simulink model "Xcvr_SSB_AM_2p5"  (Simulink 8.0)
settings: Solver=VariableStepDiscrete  SolverMode=SingleTasking  StartTime=0.0  StopTime=10  RelTol=1e-3
PreLoadFcn:
  | Fs=80e6;
  | 
  | phee=da_rom();
  | [phee_1,phee_2]=da_i2_rom();
  | 
  | Dcic=64;       % CIC decimation
  | Dfac=128;    % following DA filter decimation
  | N = 6;           %       (2^(N+1))=Dfac
  | Daudio=Dcic*Dfac;
  | Faudio=Fs/Daudio;
  | 
  | load info_filt_ssb_4
  | load Serial_Intfc_Stream_5
  | 
  | % AGC related
  | x=0.5:1/256:(1-1/256);
  | addr=(x-0.5)*256;
  | y=1./x;
values from neighbouring files (symbols this model uses):
  Serial_Interface = [0 0 0 0 0 0 0 0 0 0 0 0 ... (11390 elements, 2x5695)]    [Serial_Intfc_Stream_5.mat]
undefined symbols (not defined in the file or in its folder): get, sided, Two, xlipgetpartsetting
undefined symbols (not defined in the file): ssb_coef
libraries: xbsIndex_r4 x1307, dspsrcs4 x5, simulink x2, dspsigops x2, dspsnks4 x1
(part 10 of 11)

== system Xcvr_SSB_AM_2p5/RX Filters D=8192/Decimating Filter DC Optimized in Accumulator Plus Pipelined Stage Control. Improved dynamic  range. /D=2 Bit Serial Filter Core with Piplined RAM Based SR/ROM /Accumulator ==
  Xn + Xn-8 : Inport
  "Xn-1+ Xn-7 " : Inport  Port=2
  Xn-2 + Xn-6 : Inport  Port=3
  Xn-3 + Xn-5 : Inport  Port=4
  Xn-4 : Inport  Port=5
  Yn-2 : Inport  Port=6
  Yn-4 : Inport  Port=7
  Subtract : Inport  Port=8
  Clear : Inport  Port=9
  Round : Inport  Port=10
  AddSub : xbsIndex_r4/AddSub  mode=Addition  use_carryin=off  use_carryout=off  en=off  latency=0  precision=User Defined  arith_type="Signed  (2's comp)"  n_bits=24  bin_pt=0  quantization=Truncate  overflow=Wrap  dbl_ovrd=off  use_behavioral_HDL=off  hw_selection=Fabric  pipelined=off  use_rpm=on  block_type=addsub
      settings: block_version=9.2.00
  AddSub1 : xbsIndex_r4/AddSub  mode=Addition  use_carryin=off  use_carryout=off  en=off  latency=0  precision=User Defined  arith_type="Signed  (2's comp)"  n_bits=24  bin_pt=0  quantization=Truncate  overflow=Wrap  dbl_ovrd=off  use_behavioral_HDL=off  hw_selection=Fabric  pipelined=off  use_rpm=on  block_type=addsub
      settings: block_version=9.2.00
  Concat : xbsIndex_r4/Concat  num_inputs=8  dbl_ovrd=off  block_type=concat
      settings: block_version=9.2.00
  Convert : xbsIndex_r4/Convert  gui_display_data_type=Fixed-point  arith_type="Signed  (2's comp)"  n_bits=2  bin_pt=0  float_type=Single  exp_bits=8  fraction_bits=24  quantization=Truncate  overflow=Wrap  en=off  latency=0  dbl_ovrd=off  pipeline=off  block_type=convert
      settings: block_version=9.2.00
  ROM : xbsIndex_r4/ROM  depth=256  initVector=phee  distributed_mem=Block RAM  rst=off  init_reg=0  en=off  latency=1  gui_display_data_type=Fixed-point  arith_type="Signed  (2's comp)"  n_bits=13  bin_pt=0  preci_type=Single  exp_width=8  frac_width=24  dbl_ovrd=off  optimize=Area  use_rpm=on  block_type=sprom
      settings: block_version=9.2.00
  Register_M1 : xbsIndex_r4/Register  init=0  rst=on  en=off  dbl_ovrd=off  block_type=register
      settings: block_version=9.2.00
  Reinterpret1 : xbsIndex_r4/Reinterpret  force_arith_type=on  arith_type="Signed  (2's comp)"  force_bin_pt=on  bin_pt=0  block_type=reinterpret
      settings: infoedit="Changes signal type without altering the binary representation.   You can changed the signal between signed and unsigned, and relocate the binary point.<br><br>Hardware notes: In hardware this block costs nothing.<br><br>Example:  Suppose the input is 6 bits wide, signed, with 2 fractional bits, and the output is forced to unsigned with 0 fractional bits.  Then an input of -2.0 (1110.00 in binary 2's complement) becomes an output of 56 (111000 in binary)."  block_version=9.2.00
  Shift : xbsIndex_r4/Shift  shift_dir=Right  shift_bits=1  en=off  latency=0  precision=Full  arith_type="Signed  (2's comp)"  n_bits=18  bin_pt=0  quantization=Truncate  overflow=Wrap  dbl_ovrd=off  block_type=shift
      settings: block_version=9.2.00
  Shift1 : xbsIndex_r4/Shift  shift_dir=Left  shift_bits=10  en=off  latency=0  precision=User Defined  arith_type="Signed  (2's comp)"  n_bits=23  bin_pt=0  quantization=Truncate  overflow=Wrap  dbl_ovrd=off  block_type=shift
      settings: block_version=9.2.00
  Slice2 : xbsIndex_r4/Slice  nbits=21  boolean_output=off  mode=Lower Bit Location + Width  bit1=0  base1=MSB of Input  bit0=0  base0=LSB of Input  dbl_ovrd=off  block_type=slice
      settings: block_version=9.2.00
  Out1 : Outport
  wires:
  Subtract/1 -> Concat/1
  "Xn-1+ Xn-7 "/1 -> Concat/7
  Xn-2 + Xn-6/1 -> Concat/6
  Xn-3 + Xn-5/1 -> Concat/5
  Xn-4/1 -> Concat/4
  Yn-2/1 -> Concat/3
  Yn-4/1 -> Concat/2
  Xn + Xn-8/1 -> Concat/8
  Concat/1 -> ROM/1
  Clear/1 -> Register_M1/2
  Round/1 -> Convert/1
  ROM/1 -> Shift1/1
  Convert/1 -> AddSub1/2
  AddSub1/1 -> AddSub/2
  AddSub/1 -> Register_M1/1
  Reinterpret1/1 -> Out1/1
  Slice2/1 -> Reinterpret1/1
  Shift/1 -> AddSub/1
  Shift1/1 -> AddSub1/1
  Register_M1/1 -> Slice2/1, Shift/1

== system Xcvr_SSB_AM_2p5/RX Filters D=8192/Decimating Filter DC Optimized in Accumulator Plus Pipelined Stage Control. Improved dynamic  range. /D=2 Bit Serial Filter Core with Piplined RAM Based SR/SAD_1 ==
  A : Inport
  B : Inport  Port=2
  Clear : Inport  Port=3
  Full Adder : Subsystem
  Register : xbsIndex_r4/Register  init=0  rst=on  en=off  dbl_ovrd=off  block_type=register
      settings: block_version=9.2.00
  Sum : Outport
  wires:
  Full Adder/1(Sum) -> Sum/1
  Full Adder/2(Cout) -> Register/1
  Register/1 -> Full Adder/3(Cin)
  A/1 -> Full Adder/1(A)
  B/1 -> Full Adder/2(B)
  Clear/1 -> Register/2

== system Xcvr_SSB_AM_2p5/RX Filters D=8192/Decimating Filter DC Optimized in Accumulator Plus Pipelined Stage Control. Improved dynamic  range. /D=2 Bit Serial Filter Core with Piplined RAM Based SR/SAD_2 ==
  A : Inport
  B : Inport  Port=2
  Clear : Inport  Port=3
  Full Adder : Subsystem
  Register : xbsIndex_r4/Register  init=0  rst=on  en=off  dbl_ovrd=off  block_type=register
      settings: block_version=9.2.00
  Sum : Outport
  wires:
  Clear/1 -> Register/2
  B/1 -> Full Adder/2(B)
  A/1 -> Full Adder/1(A)
  Register/1 -> Full Adder/3(Cin)
  Full Adder/2(Cout) -> Register/1
  Full Adder/1(Sum) -> Sum/1

== system Xcvr_SSB_AM_2p5/RX Filters D=8192/Decimating Filter DC Optimized in Accumulator Plus Pipelined Stage Control. Improved dynamic  range. /D=2 Bit Serial Filter Core with Piplined RAM Based SR/SAD_3 ==
  A : Inport
  B : Inport  Port=2
  Clear : Inport  Port=3
  Full Adder : Subsystem
  Register : xbsIndex_r4/Register  init=0  rst=on  en=off  dbl_ovrd=off  block_type=register
      settings: block_version=9.2.00
  Sum : Outport
  wires:
  Full Adder/1(Sum) -> Sum/1
  Full Adder/2(Cout) -> Register/1
  Register/1 -> Full Adder/3(Cin)
  A/1 -> Full Adder/1(A)
  B/1 -> Full Adder/2(B)
  Clear/1 -> Register/2

== system Xcvr_SSB_AM_2p5/RX Filters D=8192/Decimating Filter DC Optimized in Accumulator Plus Pipelined Stage Control. Improved dynamic  range. /D=2 Bit Serial Filter Core with Piplined RAM Based SR/SAD_4 ==
  A : Inport
  B : Inport  Port=2
  Clear : Inport  Port=3
  Full Adder : Subsystem
  Register : xbsIndex_r4/Register  init=0  rst=on  en=off  dbl_ovrd=off  block_type=register
      settings: block_version=9.2.00
  Sum : Outport
  wires:
  Clear/1 -> Register/2
  B/1 -> Full Adder/2(B)
  A/1 -> Full Adder/1(A)
  Register/1 -> Full Adder/3(Cin)
  Full Adder/2(Cout) -> Register/1
  Full Adder/1(Sum) -> Sum/1

== system Xcvr_SSB_AM_2p5/RX Filters D=8192/Decimating Filter DC Optimized in Accumulator Plus Pipelined Stage Control. Improved dynamic  range. /D=2 Bit Serial Filter Core with Piplined RAM Based SR/SRA ==
  Par_In : Inport
  Shift : Inport  Port=2
  Delay : xbsIndex_r4/Delay  rst=off  infoeditControl=Selection of Reset will increase slice count due to use of real FFs and instead of SRLs  en=off  latency=1  dbl_ovrd=off  reg_retiming=off  block_type=delay
      settings: block_version=9.2.00
  Delay1 : xbsIndex_r4/Delay  rst=off  infoeditControl=Selection of Reset will increase slice count due to use of real FFs and instead of SRLs  en=off  latency=1  dbl_ovrd=off  reg_retiming=off  block_type=delay
      settings: block_version=9.2.00
  Mux : xbsIndex_r4/Mux  inputs=2  en=off  latency=0  precision=Full  arith_type=Unsigned  n_bits=16  bin_pt=14  quantization=Truncate  overflow=Wrap  dbl_ovrd=off  block_type=mux
      settings: block_version=9.2.00
  Shift1 : xbsIndex_r4/Shift  shift_dir=Right  shift_bits=1  en=off  latency=0  precision=Full  arith_type="Signed  (2's comp)"  n_bits=16  bin_pt=14  quantization=Truncate  overflow=Wrap  dbl_ovrd=off  block_type=shift
      settings: block_version=9.2.00
  Slice : xbsIndex_r4/Slice  nbits=1  boolean_output=on  mode=Lower Bit Location + Width  bit1=0  base1=MSB of Input  bit0=0  base0=LSB of Input  dbl_ovrd=off  block_type=slice
      settings: infoedit="Extracts a given range of bits from each input sample and presents it at the output.  The output type is ordinarily unsigned with binary point at zero, but can be Boolean when the slice is one bit wide.<P><P>Hardware notes: In hardware this block costs nothing."  block_version=9.2.00
  Ser_Out : Outport
  wires:
  Delay1/1 -> Ser_Out/1
  Slice/1 -> Delay1/1
  Shift/1 -> Mux/1
  Mux/1 -> Slice/1, Shift1/1
  Delay/1 -> Mux/3
  Shift1/1 -> Delay/1
  Par_In/1 -> Mux/2

== system Xcvr_SSB_AM_2p5/RX Filters D=8192/Decimating Filter DC Optimized in Accumulator Plus Pipelined Stage Control. Improved dynamic  range. /D=2 Bit Serial Filter Core with Piplined RAM Based SR/SRB ==
  Par_In : Inport
  Shift : Inport  Port=2
  Delay : xbsIndex_r4/Delay  rst=off  infoeditControl=Selection of Reset will increase slice count due to use of real FFs and instead of SRLs  en=off  latency=1  dbl_ovrd=off  reg_retiming=off  block_type=delay
      settings: block_version=9.2.00
  Delay1 : xbsIndex_r4/Delay  rst=off  infoeditControl=Selection of Reset will increase slice count due to use of real FFs and instead of SRLs  en=off  latency=1  dbl_ovrd=off  reg_retiming=off  block_type=delay
      settings: block_version=9.2.00
  Mux : xbsIndex_r4/Mux  inputs=2  en=off  latency=0  precision=Full  arith_type=Unsigned  n_bits=16  bin_pt=14  quantization=Truncate  overflow=Wrap  dbl_ovrd=off  block_type=mux
      settings: block_version=9.2.00
  Shift1 : xbsIndex_r4/Shift  shift_dir=Right  shift_bits=1  en=off  latency=0  precision=Full  arith_type="Signed  (2's comp)"  n_bits=16  bin_pt=14  quantization=Truncate  overflow=Wrap  dbl_ovrd=off  block_type=shift
      settings: block_version=9.2.00
  Slice : xbsIndex_r4/Slice  nbits=1  boolean_output=on  mode=Lower Bit Location + Width  bit1=0  base1=MSB of Input  bit0=0  base0=LSB of Input  dbl_ovrd=off  block_type=slice
      settings: infoedit="Extracts a given range of bits from each input sample and presents it at the output.  The output type is ordinarily unsigned with binary point at zero, but can be Boolean when the slice is one bit wide.<P><P>Hardware notes: In hardware this block costs nothing."  block_version=9.2.00
  Ser_Out : Outport
  wires:
  Delay1/1 -> Ser_Out/1
  Slice/1 -> Delay1/1
  Par_In/1 -> Mux/2
  Shift1/1 -> Delay/1
  Delay/1 -> Mux/3
  Mux/1 -> Shift1/1, Slice/1
  Shift/1 -> Mux/1

== system Xcvr_SSB_AM_2p5/RX Filters D=8192/Decimating Filter DC Optimized in Accumulator Plus Pipelined Stage Control. Improved dynamic  range. /D=2 Bit Serial Filter Core with Piplined RAM Based SR/SRC ==
  Par_In : Inport
  Shift : Inport  Port=2
  Delay : xbsIndex_r4/Delay  rst=off  infoeditControl=Selection of Reset will increase slice count due to use of real FFs and instead of SRLs  en=off  latency=1  dbl_ovrd=off  reg_retiming=off  block_type=delay
      settings: block_version=9.2.00
  Delay1 : xbsIndex_r4/Delay  rst=off  infoeditControl=Selection of Reset will increase slice count due to use of real FFs and instead of SRLs  en=off  latency=1  dbl_ovrd=off  reg_retiming=off  block_type=delay
      settings: block_version=9.2.00
  Mux : xbsIndex_r4/Mux  inputs=2  en=off  latency=0  precision=Full  arith_type=Unsigned  n_bits=16  bin_pt=14  quantization=Truncate  overflow=Wrap  dbl_ovrd=off  block_type=mux
      settings: block_version=9.2.00
  Shift1 : xbsIndex_r4/Shift  shift_dir=Right  shift_bits=1  en=off  latency=0  precision=Full  arith_type="Signed  (2's comp)"  n_bits=16  bin_pt=14  quantization=Truncate  overflow=Wrap  dbl_ovrd=off  block_type=shift
      settings: block_version=9.2.00
  Slice : xbsIndex_r4/Slice  nbits=1  boolean_output=on  mode=Lower Bit Location + Width  bit1=0  base1=MSB of Input  bit0=0  base0=LSB of Input  dbl_ovrd=off  block_type=slice
      settings: infoedit="Extracts a given range of bits from each input sample and presents it at the output.  The output type is ordinarily unsigned with binary point at zero, but can be Boolean when the slice is one bit wide.<P><P>Hardware notes: In hardware this block costs nothing."  block_version=9.2.00
  Ser_Out : Outport
  wires:
  Delay1/1 -> Ser_Out/1
  Slice/1 -> Delay1/1
  Shift/1 -> Mux/1
  Mux/1 -> Slice/1, Shift1/1
  Delay/1 -> Mux/3
  Shift1/1 -> Delay/1
  Par_In/1 -> Mux/2

== system Xcvr_SSB_AM_2p5/RX Filters D=8192/Decimating Filter DC Optimized in Accumulator Plus Pipelined Stage Control. Improved dynamic  range. /D=2 Bit Serial Filter Core with Piplined RAM Based SR/Timing/Control1 ==
  Start : Inport
  AddSub : xbsIndex_r4/AddSub  mode=Addition  use_carryin=off  use_carryout=off  en=off  latency=0  precision=User Defined  arith_type=Unsigned  n_bits=5  bin_pt=0  quantization=Truncate  overflow=Wrap  dbl_ovrd=off  use_behavioral_HDL=off  hw_selection=Fabric  pipelined=off  use_rpm=on  block_type=addsub
      settings: block_version=9.2.00
  Constant : xbsIndex_r4/Constant  const=26  gui_display_data_type=Fixed-point  arith_type=Unsigned  n_bits=5  bin_pt=0  preci_type=Single  exp_width=8  frac_width=24  explicit_period=off  period=1  equ=P=C  opselect=C  inp2=PCIN>>17  opr=+  inp1=P  carry=CIN  dbl_ovrd=off  block_type=constant
      settings: block_version=9.2.00
  Constant1 : xbsIndex_r4/Constant  const=1  gui_display_data_type=Fixed-point  arith_type=Unsigned  n_bits=5  bin_pt=0  preci_type=Single  exp_width=8  frac_width=24  explicit_period=off  period=1  equ=P=C  opselect=C  inp2=PCIN>>17  opr=+  inp1=P  carry=CIN  dbl_ovrd=off  block_type=constant
      settings: block_version=9.2.00
  Constant12 : xbsIndex_r4/Constant  const=2  gui_display_data_type=Fixed-point  arith_type=Unsigned  n_bits=5  bin_pt=0  preci_type=Single  exp_width=8  frac_width=24  explicit_period=off  period=1  equ=P=C  opselect=C  inp2=PCIN>>17  opr=+  inp1=P  carry=CIN  dbl_ovrd=off  block_type=constant
      settings: block_version=9.2.00
  Constant2 : xbsIndex_r4/Constant  const=0  gui_display_data_type=Fixed-point  arith_type=Unsigned  n_bits=5  bin_pt=0  preci_type=Single  exp_width=8  frac_width=24  explicit_period=off  period=1  equ=P=C  opselect=C  inp2=PCIN>>17  opr=+  inp1=P  carry=CIN  dbl_ovrd=off  block_type=constant
      settings: block_version=9.2.00
  Constant3 : xbsIndex_r4/Constant  const=0  gui_display_data_type=Fixed-point  arith_type=Unsigned  n_bits=5  bin_pt=0  preci_type=Single  exp_width=8  frac_width=24  explicit_period=off  period=1  equ=P=C  opselect=C  inp2=PCIN>>17  opr=+  inp1=P  carry=CIN  dbl_ovrd=off  block_type=constant
      settings: block_version=9.2.00
  Constant4 : xbsIndex_r4/Constant  const=1  gui_display_data_type=Fixed-point  arith_type=Unsigned  n_bits=5  bin_pt=0  preci_type=Single  exp_width=8  frac_width=24  explicit_period=off  period=1  equ=P=C  opselect=C  inp2=PCIN>>17  opr=+  inp1=P  carry=CIN  dbl_ovrd=off  block_type=constant
      settings: block_version=9.2.00
  Constant5 : xbsIndex_r4/Constant  const=25  gui_display_data_type=Fixed-point  arith_type=Unsigned  n_bits=5  bin_pt=0  preci_type=Single  exp_width=8  frac_width=24  explicit_period=off  period=1  equ=P=C  opselect=C  inp2=PCIN>>17  opr=+  inp1=P  carry=CIN  dbl_ovrd=off  block_type=constant
      settings: block_version=9.2.00
  Constant6 : xbsIndex_r4/Constant  const=23  gui_display_data_type=Fixed-point  arith_type=Unsigned  n_bits=5  bin_pt=0  preci_type=Single  exp_width=8  frac_width=24  explicit_period=off  period=1  equ=P=C  opselect=C  inp2=PCIN>>17  opr=+  inp1=P  carry=CIN  dbl_ovrd=off  block_type=constant
      settings: block_version=9.2.00
  Constant7 : xbsIndex_r4/Constant  const=2-1  gui_display_data_type=Fixed-point  arith_type=Unsigned  n_bits=5  bin_pt=0  preci_type=Single  exp_width=8  frac_width=24  explicit_period=off  period=1  equ=P=C  opselect=C  inp2=PCIN>>17  opr=+  inp1=P  carry=CIN  dbl_ovrd=off  block_type=constant
      settings: block_version=9.2.00
  Constant8 : xbsIndex_r4/Constant  const=21  gui_display_data_type=Fixed-point  arith_type=Unsigned  n_bits=5  bin_pt=0  preci_type=Single  exp_width=8  frac_width=24  explicit_period=off  period=1  equ=P=C  opselect=C  inp2=PCIN>>17  opr=+  inp1=P  carry=CIN  dbl_ovrd=off  block_type=constant
      settings: block_version=9.2.00
  Constant9 : xbsIndex_r4/Constant  const=23  gui_display_data_type=Fixed-point  arith_type=Unsigned  n_bits=5  bin_pt=0  preci_type=Single  exp_width=8  frac_width=24  explicit_period=off  period=1  equ=P=C  opselect=C  inp2=PCIN>>17  opr=+  inp1=P  carry=CIN  dbl_ovrd=off  block_type=constant
      settings: block_version=9.2.00
  Delay : xbsIndex_r4/Delay  rst=off  infoeditControl=Selection of Reset will increase slice count due to use of real FFs and instead of SRLs  en=off  latency=1  dbl_ovrd=off  reg_retiming=off  block_type=delay
      settings: block_version=9.2.00
  Logical : xbsIndex_r4/Logical  logical_function=AND  inputs=2  en=off  latency=0  precision=Full  arith_type=Unsigned  n_bits=16  bin_pt=0  align_bp=on  dbl_ovrd=off  block_type=logical
      settings: block_version=9.2.00
  Mux : xbsIndex_r4/Mux  inputs=2  en=off  latency=0  precision=Full  arith_type=Unsigned  n_bits=16  bin_pt=14  quantization=Truncate  overflow=Wrap  dbl_ovrd=off  block_type=mux
      settings: block_version=9.2.00
  Relational{,2..4,7,10} (6 alike) : xbsIndex_r4/Relational  mode=a=b  en=off  latency=0  dbl_ovrd=off  block_type=relational
      settings: block_version=9.2.00
  Relational1 : xbsIndex_r4/Relational  mode=a>b  en=off  latency=0  dbl_ovrd=off  block_type=relational
      settings: block_version=9.2.00
  Relational5 : xbsIndex_r4/Relational  mode=a>=b  en=off  latency=0  dbl_ovrd=off  block_type=relational
      settings: block_version=9.2.00
  Relational6 : xbsIndex_r4/Relational  mode=a<=b  en=off  latency=0  dbl_ovrd=off  block_type=relational
      settings: block_version=9.2.00
  S-R FF1 : Subsystem
  Run : Outport
  Clear_Adder : Outport  Port=2
  Strobe : Outport  Port=3
  Subtract : Outport  Port=4
  SR Enable : Outport  Port=5
  Round : Outport  Port=6
  Clear_Acc : Outport  Port=7
  Valid : Outport  Port=8
  wires:
  Relational4/1 -> Subtract/1
  Relational1/1 -> Run/1
  Delay/1 -> Relational5/1, Relational6/1, Relational7/1, Relational3/1, Relational2/1, AddSub/1, Relational/1, Relational1/1, Relational10/1, Relational4/1
  Relational/1 -> S-R FF1/2(Reset), Valid/1
  Constant/1 -> Relational/2
  S-R FF1/1(Q) -> Mux/1
  Start/1 -> S-R FF1/1(Set)
  Mux/1 -> Delay/1
  AddSub/1 -> Mux/3
  Constant1/1 -> AddSub/2
  Constant2/1 -> Mux/2
  Constant3/1 -> Relational1/2
  Constant4/1 -> Relational2/2
  Relational2/1 -> Clear_Adder/1
  Constant5/1 -> Relational3/2
  Relational3/1 -> Strobe/1
  Constant6/1 -> Relational4/2
  Constant7/1 -> Relational5/2
  Constant8/1 -> Relational6/2
  Relational5/1 -> Logical/1
  Relational6/1 -> Logical/2
  Logical/1 -> SR Enable/1
  Constant9/1 -> Relational7/2
  Relational7/1 -> Round/1
  Constant12/1 -> Relational10/2
  Relational10/1 -> Clear_Acc/1

== system Xcvr_SSB_AM_2p5/RX Filters D=8192/Decimating Filter DC Optimized in Accumulator Plus Pipelined Stage Control. Improved dynamic  range. /Stage Control with Pipe/Stage_Control ==
  Concat : xbsIndex_r4/Concat  num_inputs=3  dbl_ovrd=off  block_type=concat
      settings: block_version=9.2.00
  Counter : xbsIndex_r4/Counter  cnt_type=Free Running  cnt_to=Inf  operation=Up  start_count=0  cnt_by_val=1  arith_type=Unsigned  n_bits=7  bin_pt=0  load_pin=off  rst=off  en=off  explicit_period=on  period=64/Fs  dbl_ovrd=off  use_behavioral_HDL=off  implementation=Fabric  use_rpm=off  block_type=counter
      settings: block_version=9.2.00
  Logical : xbsIndex_r4/Logical  logical_function=NAND  inputs=7  en=off  latency=0  precision=Full  arith_type=Unsigned  n_bits=16  bin_pt=0  align_bp=on  dbl_ovrd=off  block_type=logical
      settings: block_version=9.2.00
  Priority_Encoder : Subsystem
  bit_0 : xbsIndex_r4/Slice  nbits=1  boolean_output=on  mode=Lower Bit Location + Width  bit1=0  base1=MSB of Input  bit0=0  base0=LSB of Input  dbl_ovrd=off  block_type=slice
      settings: infoedit="Extracts a given range of bits from each input sample and presents it at the output.  The output type is ordinarily unsigned with binary point at zero, but can be Boolean when the slice is one bit wide.<P><P>Hardware notes: In hardware this block costs nothing."  block_version=9.2.00
  bit_1 : xbsIndex_r4/Slice  nbits=1  boolean_output=on  mode=Lower Bit Location + Width  bit1=0  base1=MSB of Input  bit0=1  base0=LSB of Input  dbl_ovrd=off  block_type=slice
      settings: infoedit="Extracts a given range of bits from each input sample and presents it at the output.  The output type is ordinarily unsigned with binary point at zero, but can be Boolean when the slice is one bit wide.<P><P>Hardware notes: In hardware this block costs nothing."  block_version=9.2.00
  bit_2 : xbsIndex_r4/Slice  nbits=1  boolean_output=on  mode=Lower Bit Location + Width  bit1=0  base1=MSB of Input  bit0=2  base0=LSB of Input  dbl_ovrd=off  block_type=slice
      settings: infoedit="Extracts a given range of bits from each input sample and presents it at the output.  The output type is ordinarily unsigned with binary point at zero, but can be Boolean when the slice is one bit wide.<P><P>Hardware notes: In hardware this block costs nothing."  block_version=9.2.00
  bit_3 : xbsIndex_r4/Slice  nbits=1  boolean_output=on  mode=Lower Bit Location + Width  bit1=0  base1=MSB of Input  bit0=3  base0=LSB of Input  dbl_ovrd=off  block_type=slice
      settings: infoedit="Extracts a given range of bits from each input sample and presents it at the output.  The output type is ordinarily unsigned with binary point at zero, but can be Boolean when the slice is one bit wide.<P><P>Hardware notes: In hardware this block costs nothing."  block_version=9.2.00
  bit_4 : xbsIndex_r4/Slice  nbits=1  boolean_output=on  mode=Lower Bit Location + Width  bit1=0  base1=MSB of Input  bit0=4  base0=LSB of Input  dbl_ovrd=off  block_type=slice
      settings: infoedit="Extracts a given range of bits from each input sample and presents it at the output.  The output type is ordinarily unsigned with binary point at zero, but can be Boolean when the slice is one bit wide.<P><P>Hardware notes: In hardware this block costs nothing."  block_version=9.2.00
  bit_5 : xbsIndex_r4/Slice  nbits=1  boolean_output=on  mode=Lower Bit Location + Width  bit1=0  base1=MSB of Input  bit0=5  base0=LSB of Input  dbl_ovrd=off  block_type=slice
      settings: infoedit="Extracts a given range of bits from each input sample and presents it at the output.  The output type is ordinarily unsigned with binary point at zero, but can be Boolean when the slice is one bit wide.<P><P>Hardware notes: In hardware this block costs nothing."  block_version=9.2.00
  bit_6 : xbsIndex_r4/Slice  nbits=1  boolean_output=on  mode=Lower Bit Location + Width  bit1=0  base1=MSB of Input  bit0=6  base0=LSB of Input  dbl_ovrd=off  block_type=slice
      settings: infoedit="Extracts a given range of bits from each input sample and presents it at the output.  The output type is ordinarily unsigned with binary point at zero, but can be Boolean when the slice is one bit wide.<P><P>Hardware notes: In hardware this block costs nothing."  block_version=9.2.00
  Write_OK : Outport
  Filt_Stage : Outport  Port=2
  wires:
  bit_0/1 -> Priority_Encoder/7(In7), Logical/7
  bit_1/1 -> Priority_Encoder/6(In6), Logical/6
  bit_2/1 -> Priority_Encoder/5(In5), Logical/5
  bit_3/1 -> Priority_Encoder/4(In4), Logical/4
  bit_4/1 -> Priority_Encoder/3(In3), Logical/3
  bit_5/1 -> Priority_Encoder/2(In2), Logical/2
  bit_6/1 -> Priority_Encoder/1(In1), Logical/1
  Counter/1 -> bit_6/1, bit_0/1, bit_1/1, bit_2/1, bit_3/1, bit_4/1, bit_5/1
  Priority_Encoder/2(Out2) -> Concat/2
  Priority_Encoder/1(Out1) -> Concat/3
  Priority_Encoder/3(Out3) -> Concat/1
  Logical/1 -> Write_OK/1  "Write_OK"
  Concat/1 -> Filt_Stage/1  "Filt_Stage"

== system Xcvr_SSB_AM_2p5/SSB / AM Mod_Demod WCS/128 Tap FIR with  Writable Coefficient Store/Information_Filter_Transient_Suppressor/N_Sample_One_Shot ==
  In : Inport
  Counter : xbsIndex_r4/Counter  cnt_type=Free Running  cnt_to=Inf  operation=Up  start_count=0  cnt_by_val=1  arith_type=Unsigned  n_bits=8  bin_pt=0  load_pin=off  rst=on  en=off  explicit_period=off  period=1  dbl_ovrd=off  use_behavioral_HDL=off  implementation=Fabric  block_type=counter
      settings: block_version=12.1
  Inverter : xbsIndex_r4/Inverter  en=off  latency=0  dbl_ovrd=off  block_type=inv
      settings: block_version=12.1
  Logical : xbsIndex_r4/Logical  logical_function=OR  inputs=2  en=off  latency=0  precision=Full  arith_type=Unsigned  n_bits=16  bin_pt=0  align_bp=on  dbl_ovrd=off  block_type=logical
      settings: block_version=12.1
  N : xbsIndex_r4/Constant  const=N  gui_display_data_type=Fixed-point  arith_type=Unsigned  n_bits=8  bin_pt=0  preci_type=Single  exp_width=8  frac_width=24  explicit_period=off  period=1  equ=P=C  opselect=C  inp2=PCIN>>17  opr=+  inp1=P  carry=CIN  dbl_ovrd=off  block_type=constant
      settings: block_version=12.1
  Register : xbsIndex_r4/Register  init=0  rst=on  en=off  dbl_ovrd=off  block_type=register
      settings: block_version=12.1
  Relational : xbsIndex_r4/Relational  mode=a=b  en=off  latency=0  dbl_ovrd=off  block_type=relational
      settings: block_version=12.1
  Out : Outport
  wires:
  Logical/1 -> Register/1, Out/1
  Register/1 -> Logical/2, Inverter/1
  In/1 -> Logical/1
  Counter/1 -> Relational/1
  N/1 -> Relational/2
  Relational/1 -> Register/2
  Inverter/1 -> Counter/1

== system Xcvr_SSB_AM_2p5/Serial Interface1/Serial_in_Parallel_out/Serial2Par/Subsystem ==
  Sin : Inport
  Ena : Inport  Port=2
  Concat : xbsIndex_r4/Concat  num_inputs=8  dbl_ovrd=off  block_type=concat
      settings: block_version=9.2.00
  Register{1..8} (8 alike) : xbsIndex_r4/Register  init=0  rst=off  en=on  dbl_ovrd=off  block_type=register
      settings: block_version=9.2.00
  Out_8b : Outport
  Sout : Outport  Port=2
  wires:
  Ena/1 -> Register8/2, Register7/2, Register6/2, Register5/2, Register4/2, Register3/2, Register2/2, Register1/2
  Register2/1 -> Register3/1, Concat/7
  Register3/1 -> Register4/1, Concat/6
  Register4/1 -> Register5/1, Concat/5
  Register5/1 -> Register6/1, Concat/4
  Register6/1 -> Register7/1, Concat/3
  Register7/1 -> Register8/1, Concat/2
  Register8/1 -> Concat/1, Sout/1
  Concat/1 -> Out_8b/1
  Register1/1 -> Concat/8, Register2/1
  Sin/1 -> Register1/1

== system Xcvr_SSB_AM_2p5/Serial Interface1/Serial_in_Parallel_out/Serial2Par/Subsystem1 ==
  Sin : Inport
  Ena : Inport  Port=2
  Concat : xbsIndex_r4/Concat  num_inputs=8  dbl_ovrd=off  block_type=concat
      settings: block_version=9.2.00
  Register{1..8} (8 alike) : xbsIndex_r4/Register  init=0  rst=off  en=on  dbl_ovrd=off  block_type=register
      settings: block_version=9.2.00
  Out_8b : Outport
  Sout : Outport  Port=2
  wires:
  Sin/1 -> Register1/1
  Concat/1 -> Out_8b/1
  Register8/1 -> Sout/1, Concat/1
  Register7/1 -> Concat/2, Register8/1
  Register6/1 -> Concat/3, Register7/1
  Register5/1 -> Concat/4, Register6/1
  Register4/1 -> Concat/5, Register5/1
  Register3/1 -> Concat/6, Register4/1
  Register2/1 -> Concat/7, Register3/1
  Register1/1 -> Concat/8, Register2/1
  Ena/1 -> Register2/2, Register3/2, Register4/2, Register5/2, Register6/2, Register7/2, Register8/2, Register1/2

== system Xcvr_SSB_AM_2p5/Serial Interface1/Serial_in_Parallel_out/Serial2Par/Subsystem2 ==
  Sin : Inport
  Ena : Inport  Port=2
  Concat : xbsIndex_r4/Concat  num_inputs=8  dbl_ovrd=off  block_type=concat
      settings: block_version=9.2.00
  Register{1..8} (8 alike) : xbsIndex_r4/Register  init=0  rst=off  en=on  dbl_ovrd=off  block_type=register
      settings: block_version=9.2.00
  Out_8b : Outport
  Sout : Outport  Port=2
  wires:
  Ena/1 -> Register1/2, Register8/2, Register7/2, Register6/2, Register5/2, Register4/2, Register3/2, Register2/2
  Register1/1 -> Register2/1, Concat/8
  Register2/1 -> Register3/1, Concat/7
  Register3/1 -> Register4/1, Concat/6
  Register4/1 -> Register5/1, Concat/5
  Register5/1 -> Register6/1, Concat/4
  Register6/1 -> Register7/1, Concat/3
  Register7/1 -> Register8/1, Concat/2
  Register8/1 -> Concat/1, Sout/1
  Concat/1 -> Out_8b/1
  Sin/1 -> Register1/1

== system Xcvr_SSB_AM_2p5/Serial Interface1/Serial_in_Parallel_out/Serial2Par/Subsystem3 ==
  Sin : Inport
  Ena : Inport  Port=2
  Concat : xbsIndex_r4/Concat  num_inputs=8  dbl_ovrd=off  block_type=concat
      settings: block_version=9.2.00
  Register{1..8} (8 alike) : xbsIndex_r4/Register  init=0  rst=off  en=on  dbl_ovrd=off  block_type=register
      settings: block_version=9.2.00
  Out_8b : Outport
  Sout : Outport  Port=2
  wires:
  Sin/1 -> Register1/1
  Concat/1 -> Out_8b/1
  Register8/1 -> Sout/1, Concat/1
  Register7/1 -> Concat/2, Register8/1
  Register6/1 -> Concat/3, Register7/1
  Register5/1 -> Concat/4, Register6/1
  Register4/1 -> Concat/5, Register5/1
  Register3/1 -> Concat/6, Register4/1
  Register2/1 -> Concat/7, Register3/1
  Register1/1 -> Concat/8, Register2/1
  Ena/1 -> Register2/2, Register3/2, Register4/2, Register5/2, Register6/2, Register7/2, Register8/2, Register1/2

== system Xcvr_SSB_AM_2p5/TX Filters I=8192/Control/Stage_Control/Priority_Encoder ==
  In1 : Inport
  In2 : Inport  Port=2
  In3 : Inport  Port=3
  In4 : Inport  Port=4
  In5 : Inport  Port=5
  In6 : Inport  Port=6
  In7 : Inport  Port=7
  Inverter{,1..6} (7 alike) : xbsIndex_r4/Inverter  en=off  latency=0  dbl_ovrd=off  block_type=inv
      settings: block_version=9.2.00
  Logical : xbsIndex_r4/Logical  logical_function=AND  inputs=4  en=off  latency=0  precision=Full  arith_type=Unsigned  n_bits=16  bin_pt=0  align_bp=on  dbl_ovrd=off  block_type=logical
      settings: block_version=9.2.00
  Logical1 : xbsIndex_r4/Logical  logical_function=NOR  inputs=4  en=off  latency=0  precision=Full  arith_type=Unsigned  n_bits=16  bin_pt=0  align_bp=on  dbl_ovrd=off  block_type=logical
      settings: block_version=9.2.00
  Logical2 : xbsIndex_r4/Logical  logical_function=AND  inputs=3  en=off  latency=0  precision=Full  arith_type=Unsigned  n_bits=16  bin_pt=0  align_bp=on  dbl_ovrd=off  block_type=logical
      settings: block_version=9.2.00
  Logical3 : xbsIndex_r4/Logical  logical_function=AND  inputs=2  en=off  latency=0  precision=Full  arith_type=Unsigned  n_bits=16  bin_pt=0  align_bp=on  dbl_ovrd=off  block_type=logical
      settings: block_version=9.2.00
  Logical4 : xbsIndex_r4/Logical  logical_function=AND  inputs=3  en=off  latency=0  precision=Full  arith_type=Unsigned  n_bits=16  bin_pt=0  align_bp=on  dbl_ovrd=off  block_type=logical
      settings: block_version=9.2.00
  Logical5 : xbsIndex_r4/Logical  logical_function=AND  inputs=3  en=off  latency=0  precision=Full  arith_type=Unsigned  n_bits=16  bin_pt=0  align_bp=on  dbl_ovrd=off  block_type=logical
      settings: block_version=9.2.00
  Logical6 : xbsIndex_r4/Logical  logical_function=NOR  inputs=4  en=off  latency=0  precision=Full  arith_type=Unsigned  n_bits=16  bin_pt=0  align_bp=on  dbl_ovrd=off  block_type=logical
      settings: block_version=9.2.00
  Logical7 : xbsIndex_r4/Logical  logical_function=NOR  inputs=4  en=off  latency=0  precision=Full  arith_type=Unsigned  n_bits=16  bin_pt=0  align_bp=on  dbl_ovrd=off  block_type=logical
      settings: block_version=9.2.00
  Out1 : Outport
  Out2 : Outport  Port=2
  Out3 : Outport  Port=3
  wires:
  Logical7/1 -> Out3/1
  Logical6/1 -> Out2/1
  In7/1 -> Inverter6/1
  Logical1/1 -> Out1/1
  In3/1 -> Inverter2/1
  In1/1 -> Inverter/1
  Inverter3/1 -> Logical7/1
  Inverter4/1 -> Logical3/1, Logical7/2
  Inverter6/1 -> Logical1/4, Logical6/4, Logical7/4
  Inverter5/1 -> Logical7/3, Logical6/3
  Inverter1/1 -> Logical4/1
  Inverter2/1 -> Logical5/1, Logical2/1
  In6/1 -> Logical3/2, Logical2/3, Logical/4, Inverter5/1
  In5/1 -> Logical5/3, Logical4/3, Inverter4/1
  In4/1 -> Logical5/2, Logical4/2, Logical2/2, Logical/3, Inverter3/1
  In2/1 -> Logical/2, Inverter1/1
  Logical5/1 -> Logical6/2
  Logical4/1 -> Logical6/1
  Logical3/1 -> Logical1/3
  Logical2/1 -> Logical1/2
  Logical/1 -> Logical1/1
  Inverter/1 -> Logical/1

== system Xcvr_SSB_AM_2p5/TX Filters I=8192/Interp_Core/RAM Based SR/Bit-Extraction ==
  In1 : Inport
  B0 : xbsIndex_r4/Slice  nbits=1  boolean_output=on  mode=Lower Bit Location + Width  bit1=0  base1=MSB of Input  bit0=0  base0=LSB of Input  dbl_ovrd=off  block_type=slice
      settings: infoedit="Extracts a given range of bits from each input sample and presents it at the output.  The output type is ordinarily unsigned with binary point at zero, but can be Boolean when the slice is one bit wide.<P><P>Hardware notes: In hardware this block costs nothing."  block_version=9.2.00
  B1 : xbsIndex_r4/Slice  nbits=1  boolean_output=on  mode=Lower Bit Location + Width  bit1=0  base1=MSB of Input  bit0=1  base0=LSB of Input  dbl_ovrd=off  block_type=slice
      settings: infoedit="Extracts a given range of bits from each input sample and presents it at the output.  The output type is ordinarily unsigned with binary point at zero, but can be Boolean when the slice is one bit wide.<P><P>Hardware notes: In hardware this block costs nothing."  block_version=9.2.00
  B2 : xbsIndex_r4/Slice  nbits=1  boolean_output=on  mode=Lower Bit Location + Width  bit1=0  base1=MSB of Input  bit0=2  base0=LSB of Input  dbl_ovrd=off  block_type=slice
      settings: infoedit="Extracts a given range of bits from each input sample and presents it at the output.  The output type is ordinarily unsigned with binary point at zero, but can be Boolean when the slice is one bit wide.<P><P>Hardware notes: In hardware this block costs nothing."  block_version=9.2.00
  B3 : xbsIndex_r4/Slice  nbits=1  boolean_output=on  mode=Lower Bit Location + Width  bit1=0  base1=MSB of Input  bit0=3  base0=LSB of Input  dbl_ovrd=off  block_type=slice
      settings: infoedit="Extracts a given range of bits from each input sample and presents it at the output.  The output type is ordinarily unsigned with binary point at zero, but can be Boolean when the slice is one bit wide.<P><P>Hardware notes: In hardware this block costs nothing."  block_version=9.2.00
  B4 : xbsIndex_r4/Slice  nbits=1  boolean_output=on  mode=Lower Bit Location + Width  bit1=0  base1=MSB of Input  bit0=4  base0=LSB of Input  dbl_ovrd=off  block_type=slice
      settings: infoedit="Extracts a given range of bits from each input sample and presents it at the output.  The output type is ordinarily unsigned with binary point at zero, but can be Boolean when the slice is one bit wide.<P><P>Hardware notes: In hardware this block costs nothing."  block_version=9.2.00
  B5 : xbsIndex_r4/Slice  nbits=1  boolean_output=on  mode=Lower Bit Location + Width  bit1=0  base1=MSB of Input  bit0=5  base0=LSB of Input  dbl_ovrd=off  block_type=slice
      settings: infoedit="Extracts a given range of bits from each input sample and presents it at the output.  The output type is ordinarily unsigned with binary point at zero, but can be Boolean when the slice is one bit wide.<P><P>Hardware notes: In hardware this block costs nothing."  block_version=9.2.00
  b0 : Outport
  b1 : Outport  Port=2
  b2 : Outport  Port=3
  b3 : Outport  Port=4
  b4 : Outport  Port=5
  b5 : Outport  Port=6
  wires:
  B5/1 -> b5/1
  B4/1 -> b4/1
  B3/1 -> b3/1
  B2/1 -> b2/1
  B1/1 -> b1/1
  B0/1 -> b0/1
  In1/1 -> B3/1, B0/1, B1/1, B2/1, B4/1, B5/1

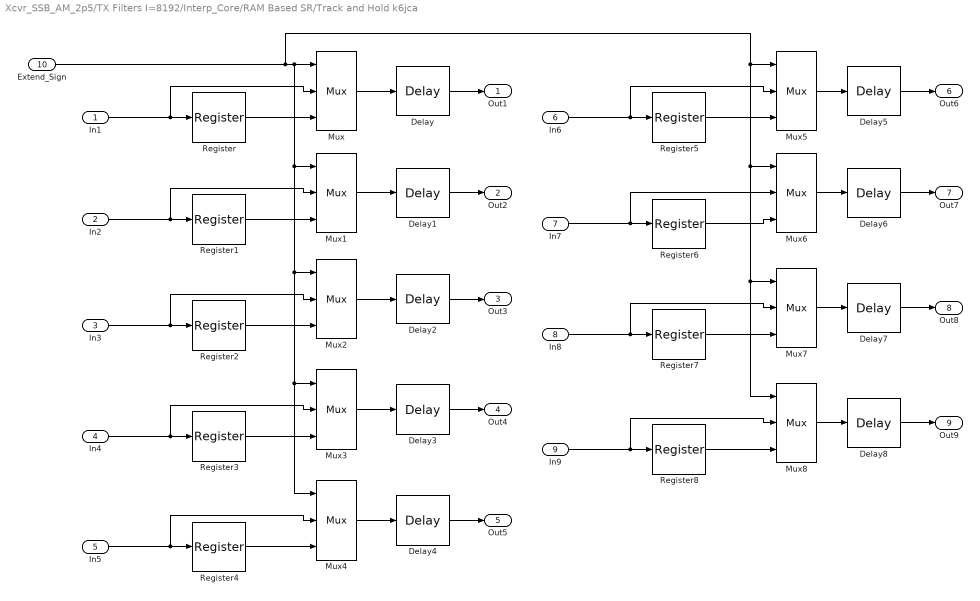
== system Xcvr_SSB_AM_2p5/TX Filters I=8192/Interp_Core/RAM Based SR/Track and Hold k6jca ==
  In1 : Inport
  In2 : Inport  Port=2
  In3 : Inport  Port=3
  In4 : Inport  Port=4
  In5 : Inport  Port=5
  In6 : Inport  Port=6
  In7 : Inport  Port=7
  In8 : Inport  Port=8
  In9 : Inport  Port=9
  Extend_Sign : Inport  Port=10
  Delay{,1..8} (9 alike) : xbsIndex_r4/Delay  rst=off  infoeditControl=Selection of Reset will increase slice count due to use of real FFs and instead of SRLs  en=off  latency=1  dbl_ovrd=off  reg_retiming=off  block_type=delay
      settings: block_version=12.2
  Mux{,1..8} (9 alike) : xbsIndex_r4/Mux  inputs=2  en=off  latency=0  precision=Full  arith_type=Unsigned  n_bits=16  bin_pt=14  quantization=Truncate  overflow=Wrap  dbl_ovrd=off  block_type=mux
      settings: block_version=12.2
  Register{,1..8} (9 alike) : xbsIndex_r4/Register  init=0  rst=off  en=off  dbl_ovrd=off  block_type=register
      settings: block_version=12.2
  Out1 : Outport
  Out2 : Outport  Port=2
  Out3 : Outport  Port=3
  Out4 : Outport  Port=4
  Out5 : Outport  Port=5
  Out6 : Outport  Port=6
  Out7 : Outport  Port=7
  Out8 : Outport  Port=8
  Out9 : Outport  Port=9
  wires:
  Register/1 -> Mux/3
  In1/1 -> Register/1, Mux/2
  Extend_Sign/1 -> Mux/1, Mux1/1, Mux2/1, Mux4/1, Mux3/1, Mux5/1, Mux8/1, Mux7/1, Mux6/1
  Register1/1 -> Mux1/3
  In2/1 -> Register1/1, Mux1/2
  Register2/1 -> Mux2/3
  In3/1 -> Register2/1, Mux2/2
  Register3/1 -> Mux3/3
  In4/1 -> Register3/1, Mux3/2
  Register4/1 -> Mux4/3
  In5/1 -> Register4/1, Mux4/2
  Register5/1 -> Mux5/3
  In6/1 -> Register5/1, Mux5/2
  Register6/1 -> Mux6/3
  In7/1 -> Register6/1, Mux6/2
  Register7/1 -> Mux7/3
  In8/1 -> Register7/1, Mux7/2
  Register8/1 -> Mux8/3
  In9/1 -> Register8/1, Mux8/2
  Mux/1 -> Delay/1
  Delay/1 -> Out1/1
  Mux1/1 -> Delay1/1
  Delay1/1 -> Out2/1
  Mux2/1 -> Delay2/1
  Delay2/1 -> Out3/1
  Mux3/1 -> Delay3/1
  Delay3/1 -> Out4/1
  Mux4/1 -> Delay4/1
  Delay4/1 -> Out5/1
  Mux5/1 -> Delay5/1
  Mux6/1 -> Delay6/1
  Delay5/1 -> Out6/1
  Delay6/1 -> Out7/1
  Mux7/1 -> Delay7/1
  Delay7/1 -> Out8/1
  Mux8/1 -> Delay8/1
  Delay8/1 -> Out9/1

== system Xcvr_SSB_AM_2p5/TX Filters I=8192/Interp_Core/SAD_1/Full Adder ==
  note: Full Adder Logic
  A : Inport
  B : Inport  Port=2
  Cin : Inport  Port=3
  Logical : xbsIndex_r4/Logical  logical_function=AND  inputs=2  en=off  latency=0  precision=Full  arith_type=Unsigned  n_bits=16  bin_pt=0  align_bp=on  dbl_ovrd=off  block_type=logical
      settings: block_version=9.2.00
  Logical1 : xbsIndex_r4/Logical  logical_function=AND  inputs=2  en=off  latency=0  precision=Full  arith_type=Unsigned  n_bits=16  bin_pt=0  align_bp=on  dbl_ovrd=off  block_type=logical
      settings: block_version=9.2.00
  Logical2 : xbsIndex_r4/Logical  logical_function=OR  inputs=2  en=off  latency=0  precision=Full  arith_type=Unsigned  n_bits=16  bin_pt=0  align_bp=on  dbl_ovrd=off  block_type=logical
      settings: block_version=9.2.00
  Logical3 : xbsIndex_r4/Logical  logical_function=XOR  inputs=2  en=off  latency=0  precision=Full  arith_type=Unsigned  n_bits=16  bin_pt=0  align_bp=on  dbl_ovrd=off  block_type=logical
      settings: block_version=9.2.00
  Logical4 : xbsIndex_r4/Logical  logical_function=XOR  inputs=2  en=off  latency=0  precision=Full  arith_type=Unsigned  n_bits=16  bin_pt=0  align_bp=on  dbl_ovrd=off  block_type=logical
      settings: block_version=9.2.00
  Sum : Outport
  Cout : Outport  Port=2
  wires:
  Logical2/1 -> Cout/1  "Cout"
  Logical4/1 -> Sum/1  "Sout"
  Logical1/1 -> Logical2/1
  Logical/1 -> Logical2/2
  A/1 -> Logical3/1, Logical/1
  B/1 -> Logical3/2, Logical/2
  Cin/1 -> Logical4/2, Logical1/1
  Logical3/1 -> Logical4/1, Logical1/2

== system Xcvr_SSB_AM_2p5/TX Filters I=8192/Interp_Core/SAD_2/Full Adder ==
  note: Full Adder Logic
  A : Inport
  B : Inport  Port=2
  Cin : Inport  Port=3
  Logical : xbsIndex_r4/Logical  logical_function=AND  inputs=2  en=off  latency=0  precision=Full  arith_type=Unsigned  n_bits=16  bin_pt=0  align_bp=on  dbl_ovrd=off  block_type=logical
      settings: block_version=9.2.00
  Logical1 : xbsIndex_r4/Logical  logical_function=AND  inputs=2  en=off  latency=0  precision=Full  arith_type=Unsigned  n_bits=16  bin_pt=0  align_bp=on  dbl_ovrd=off  block_type=logical
      settings: block_version=9.2.00
  Logical2 : xbsIndex_r4/Logical  logical_function=OR  inputs=2  en=off  latency=0  precision=Full  arith_type=Unsigned  n_bits=16  bin_pt=0  align_bp=on  dbl_ovrd=off  block_type=logical
      settings: block_version=9.2.00
  Logical3 : xbsIndex_r4/Logical  logical_function=XOR  inputs=2  en=off  latency=0  precision=Full  arith_type=Unsigned  n_bits=16  bin_pt=0  align_bp=on  dbl_ovrd=off  block_type=logical
      settings: block_version=9.2.00
  Logical4 : xbsIndex_r4/Logical  logical_function=XOR  inputs=2  en=off  latency=0  precision=Full  arith_type=Unsigned  n_bits=16  bin_pt=0  align_bp=on  dbl_ovrd=off  block_type=logical
      settings: block_version=9.2.00
  Sum : Outport
  Cout : Outport  Port=2
  wires:
  Logical3/1 -> Logical1/2, Logical4/1
  Cin/1 -> Logical1/1, Logical4/2
  B/1 -> Logical/2, Logical3/2
  A/1 -> Logical/1, Logical3/1
  Logical/1 -> Logical2/2
  Logical1/1 -> Logical2/1
  Logical4/1 -> Sum/1  "Sout"
  Logical2/1 -> Cout/1  "Cout"

== system Xcvr_SSB_AM_2p5/TX Filters I=8192/Interp_Core/SAD_3/Full Adder ==
  note: Full Adder Logic
  A : Inport
  B : Inport  Port=2
  Cin : Inport  Port=3
  Logical : xbsIndex_r4/Logical  logical_function=AND  inputs=2  en=off  latency=0  precision=Full  arith_type=Unsigned  n_bits=16  bin_pt=0  align_bp=on  dbl_ovrd=off  block_type=logical
      settings: block_version=9.2.00
  Logical1 : xbsIndex_r4/Logical  logical_function=AND  inputs=2  en=off  latency=0  precision=Full  arith_type=Unsigned  n_bits=16  bin_pt=0  align_bp=on  dbl_ovrd=off  block_type=logical
      settings: block_version=9.2.00
  Logical2 : xbsIndex_r4/Logical  logical_function=OR  inputs=2  en=off  latency=0  precision=Full  arith_type=Unsigned  n_bits=16  bin_pt=0  align_bp=on  dbl_ovrd=off  block_type=logical
      settings: block_version=9.2.00
  Logical3 : xbsIndex_r4/Logical  logical_function=XOR  inputs=2  en=off  latency=0  precision=Full  arith_type=Unsigned  n_bits=16  bin_pt=0  align_bp=on  dbl_ovrd=off  block_type=logical
      settings: block_version=9.2.00
  Logical4 : xbsIndex_r4/Logical  logical_function=XOR  inputs=2  en=off  latency=0  precision=Full  arith_type=Unsigned  n_bits=16  bin_pt=0  align_bp=on  dbl_ovrd=off  block_type=logical
      settings: block_version=9.2.00
  Sum : Outport
  Cout : Outport  Port=2
  wires:
  Logical2/1 -> Cout/1  "Cout"
  Logical4/1 -> Sum/1  "Sout"
  Logical1/1 -> Logical2/1
  Logical/1 -> Logical2/2
  A/1 -> Logical3/1, Logical/1
  B/1 -> Logical3/2, Logical/2
  Cin/1 -> Logical4/2, Logical1/1
  Logical3/1 -> Logical4/1, Logical1/2

== system Xcvr_SSB_AM_2p5/TX Filters I=8192/Interp_Core/SAD_4/Full Adder ==
  note: Full Adder Logic
  A : Inport
  B : Inport  Port=2
  Cin : Inport  Port=3
  Logical : xbsIndex_r4/Logical  logical_function=AND  inputs=2  en=off  latency=0  precision=Full  arith_type=Unsigned  n_bits=16  bin_pt=0  align_bp=on  dbl_ovrd=off  block_type=logical
      settings: block_version=9.2.00
  Logical1 : xbsIndex_r4/Logical  logical_function=AND  inputs=2  en=off  latency=0  precision=Full  arith_type=Unsigned  n_bits=16  bin_pt=0  align_bp=on  dbl_ovrd=off  block_type=logical
      settings: block_version=9.2.00
  Logical2 : xbsIndex_r4/Logical  logical_function=OR  inputs=2  en=off  latency=0  precision=Full  arith_type=Unsigned  n_bits=16  bin_pt=0  align_bp=on  dbl_ovrd=off  block_type=logical
      settings: block_version=9.2.00
  Logical3 : xbsIndex_r4/Logical  logical_function=XOR  inputs=2  en=off  latency=0  precision=Full  arith_type=Unsigned  n_bits=16  bin_pt=0  align_bp=on  dbl_ovrd=off  block_type=logical
      settings: block_version=9.2.00
  Logical4 : xbsIndex_r4/Logical  logical_function=XOR  inputs=2  en=off  latency=0  precision=Full  arith_type=Unsigned  n_bits=16  bin_pt=0  align_bp=on  dbl_ovrd=off  block_type=logical
      settings: block_version=9.2.00
  Sum : Outport
  Cout : Outport  Port=2
  wires:
  Logical3/1 -> Logical1/2, Logical4/1
  Cin/1 -> Logical1/1, Logical4/2
  B/1 -> Logical/2, Logical3/2
  A/1 -> Logical/1, Logical3/1
  Logical/1 -> Logical2/2
  Logical1/1 -> Logical2/1
  Logical4/1 -> Sum/1  "Sout"
  Logical2/1 -> Cout/1  "Cout"

== system Xcvr_SSB_AM_2p5/TX Filters I=8192/Interp_Core/Timing/Control1/S-R FF1 ==
  Set : Inport
  Reset : Inport  Port=2
  Logical : xbsIndex_r4/Logical  logical_function=OR  inputs=2  en=off  latency=0  precision=Full  arith_type=Unsigned  n_bits=16  bin_pt=0  align_bp=on  dbl_ovrd=off  block_type=logical
      settings: block_version=VER_STRING_GOES_HERE
  Register : xbsIndex_r4/Register  init=0  rst=on  en=off  dbl_ovrd=off  block_type=register
      settings: block_version=VER_STRING_GOES_HERE
  Q : Outport
  wires:
  Reset/1 -> Register/2
  Set/1 -> Logical/2
  Register/1 -> Logical/1
  Logical/1 -> Q/1, Register/1
